simulink model "RuleBasedControlTest"  (R2012b)
settings: Solver=ode1  StartTime=0.0  StopTime=Inf  FixedStep=0.001  RelTol=1e-3
PostLoadFcn:
  | , if any(exist('dsrtsu_mdlpostloadfcn', 'file') == [2, 3, 6]), try dsrtsu_mdlpostloadfcn('Execute', bdroot); catch fprintf('Error in PostLoadFcn (dsrtsu_mdlpostloadfcn) for model "%s":\n %s\n', bdroot, lasterr); end, end,
undefined symbols (not defined in the file or in its folder): RuleBasedControlHESSPowerValues, RuleBasedControlLUTValues, RuleBasedControlUCVoltageValues
settings Model: DSRTSU_INTERNAL_RTI_VER=430  DSRTSU_INTERNAL_RTI_TYPE=rti1103  DSRTSU_INTERNAL_RTIFPGA=20  BufferReuse=off  Creator=Raghav  LastModifiedBy=Raghav
settings OptimizationCC: BlockReduction=off  OptimizeBlockIOStorage=off  BufferReuse=off  ExpressionFolding=off  LocalBlockOutputs=off
settings HardwareCC: ProdIntDivRoundTo=Zero  ProdEndianess=BigEndian  ProdHWDeviceType=Generic->Custom  TargetIntDivRoundTo=Zero  TargetEndianess=BigEndian  TargetHWDeviceType=Generic->Custom
settings RTWCC: SystemTargetFile=rti1103.tlc  MakeCommand=make_rti  TemplateMakefile=rti1103.tmf  Description=dSPACE DS1103 Hardware Platform  ProcessScript=rti1103_make_rtw_hook
settings STFCustomTargetCC: CodeReplacementLibrary=ANSI_C  ParMdlRefBuildCompliant=on  GeneratePreprocessorConditionals=Disable all  MatFileLogging=on  SystemTargetFile=rti1103.tlc
settings GRTTargetCC: CompOptLevelCompliant=off  ConcurrentExecutionCompliant=off  CombineOutputUpdateFcns=off  GRTInterface=on  ExtModeMexFile=noextcomm

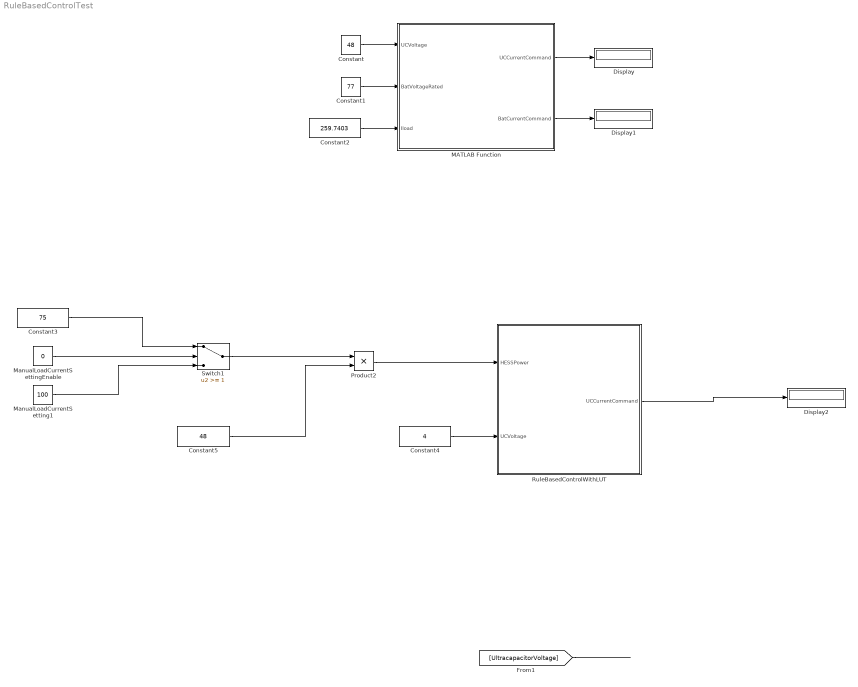
== system RuleBasedControlTest ==
  Constant : Constant  Value=48
  Constant1 : Constant  Value=77
  Constant2 : Constant  Value=259.7403
  Constant3 : Constant  Value=75
  Constant4 : Constant  Value=4
  Constant5 : Constant  Value=48
  Display : Display
  Display1 : Display
  Display2 : Display
  MATLAB Function : MATLAB Function  TreatAsAtomicUnit=on
  ManualLoadCurrentSetting1 : Constant  Value=100  SampleTime=-1
  ManualLoadCurrentSettingEnable : Constant  Value=0  SampleTime=-1
  Product2 : Product  RndMeth=Zero
  RuleBasedControlWithLUT : Subsystem
  Switch1 : Switch  Threshold=1  OutDataTypeStr=Inherit: Inherit via back propagation
  wires:
  Constant/1 -> MATLAB Function/1(UCVoltage)
  Constant1/1 -> MATLAB Function/2(BatVoltageRated)
  Constant2/1 -> MATLAB Function/3(Iload)
  MATLAB Function/1(UCCurrentCommand) -> Display/1
  MATLAB Function/2(BatCurrentCommand) -> Display1/1
  Constant4/1 -> RuleBasedControlWithLUT/2(UCVoltage)
  RuleBasedControlWithLUT/1(UCCurrentCommand) -> Display2/1
  [UltracapacitorVoltage] -> ?
  Constant5/1 -> Product2/2
  Product2/1 -> RuleBasedControlWithLUT/1(HESSPower)
  Switch1/1 -> Product2/1
  Constant3/1 -> Switch1/1
  ManualLoadCurrentSettingEnable/1 -> Switch1/2
  ManualLoadCurrentSetting1/1 -> Switch1/3

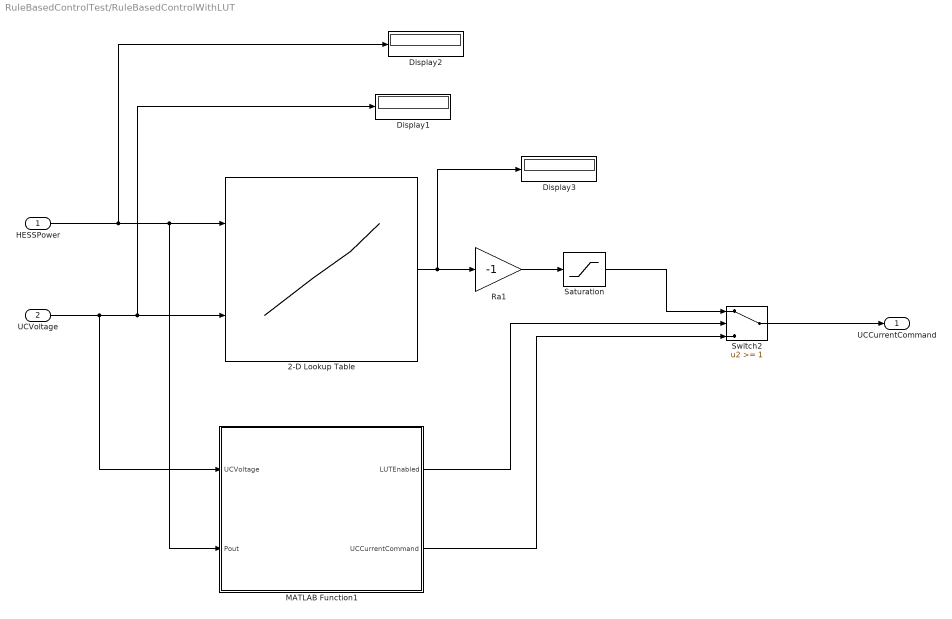
== system RuleBasedControlTest/RuleBasedControlWithLUT ==
  HESSPower : Inport
  UCVoltage : Inport  Port=2
  2-D Lookup Table : Lookup_n-D  BreakpointsForDimension1=RuleBasedControlHESSPowerValues  BreakpointsForDimension2=RuleBasedControlUCVoltageValues  BreakpointsForDimension1Min=0  BreakpointsForDimension1Max=20000  Table=RuleBasedControlLUTValues  RndMeth=Simplest  InputSameDT=on
  Display1 : Display
  Display2 : Display
  Display3 : Display
  MATLAB Function1 : MATLAB Function  TreatAsAtomicUnit=on
  Ra1 : Gain  Gain=-1
  Saturation : Saturate  UpperLimit=0  LowerLimit=-200
  Switch2 : Switch  Threshold=1  OutDataTypeStr=Inherit: Inherit via back propagation
  UCCurrentCommand : Outport
  wires:
  HESSPower/1 -> Display2/1, MATLAB Function1/2(Pout), 2-D Lookup Table/1
  MATLAB Function1/1(LUTEnabled) -> Switch2/2
  Switch2/1 -> UCCurrentCommand/1
  UCVoltage/1 -> MATLAB Function1/1(UCVoltage), Display1/1, 2-D Lookup Table/2
  MATLAB Function1/2(UCCurrentCommand) -> Switch2/3
  2-D Lookup Table/1 -> Display3/1, Ra1/1
  Ra1/1 -> Saturation/1
  Saturation/1 -> Switch2/1

== matlab function RuleBasedControlTest/MATLAB Function ==
  data: UCVoltage input; UCCurrentCommand output; BatVoltageRated input; Iload input; BatCurrentCommand output
function [UCCurrentCommand, BatCurrentCommand] = fcn(UCVoltage, BatVoltageRated, Iload)

Rb = 4*2.8e-3; % battery resistance
Ruc = 5.5e-3; % ultracap resistance
eff_dcdc = 0.95; % dcdc converter efficiency - constant approximation

% convention expected
% Iload +ve - Load is drawing power
% Iload -ve - Load is sourcing power
Pout = BatVoltageRated * Iload;

if Pout>=0
    num_array = zeros(1,3);
    num_array(1) = Rb * BatVoltageRated * UCVoltage^2;
    num_array(2) = eff_dcdc * Ruc * BatVoltageRated^3;
    num_array(3) = -BatVoltageRated * sqrt( eff_dcdc * (Ruc*eff_dcdc*BatVoltageRated^2+Rb*UCVoltage^2) * (Ruc*BatVoltageRated^2+Rb*eff_dcdc*UCVoltage^2-4*Pout*Rb*Ruc) );

    den_array = zeros(1,2);
    den_array(1) = 2*Rb^2*UCVoltage^2;
    den_array(2) = 2*eff_dcdc*Ruc*Rb*BatVoltageRated^2;

    num = sum(num_array);
    den = sum(den_array);
    BatCurrentCommand = num/den;
    
    BatPowerCommand = (BatVoltageRated - BatCurrentCommand*Rb) * BatCurrentCommand;
    UCPowerCommand = (Pout - BatPowerCommand) / eff_dcdc;
    UCCurrentCommand = UCPowerCommand/UCVoltage;

    % command sign convention in Phil Kollmeyer's formula is opposite to the one used in this controls setup
    % THIS controls setup uses
    % a) Positive Current Command for Charging the Ultracap (discharging the
    % battery)
    % b) Negative Current Command for Discharging the Utracap (charging the
    % battery)
    UCCurrentCommand = -UCCurrentCommand;
    
    % If formula asks to charge Ultracap when load is drawing power
    % Most efficient to not do anything
    if UCCurrentCommand>0
        UCCurrentCommand = 0;
    end
    
else
    PowerShareRatio = 0.8;
    PtoUC = -Pout*PowerShareRatio; % Ultracap must draw power, so polarity is reversed
    UCCurrentCommand = PtoUC/BatVoltageRated;
    
    BatCurrentCommand = 0;
end

== matlab function RuleBasedControlTest/RuleBasedControlWithLUT/MATLAB Function1 ==
  data: LUTEnabled output; UCCurrentCommand output; UCVoltage input; Pout input
function [LUTEnabled, UCCurrentCommand] = fcn(UCVoltage, Pout)

if Pout>=0
    LUTEnabled = 1;
    UCCurrentCommand = 0;
    
else
    LUTEnabled = 0;
    
    PowerShareRatio = 0.8;
    PtoUC = -Pout*PowerShareRatio; % Ultracap must draw power, so polarity is reversed
    UCCurrentCommand = PtoUC/UCVoltage;
end
